simulink library "LUT_Susp_Lib"  (R2023b)
settings: Solver=VariableStepAuto  StartTime=0.0  StopTime=10.0  RelTol=1e-3
undefined symbols (not defined in the file or in its folder): Compliance, hp_wheel_ctr, JUnsprungMass, mUnsprungMass, spring_f, spring_x, Susp, Visual
libraries: nesl_utility x12, sm_lib x5, linkage_bushing_6DOF_lib x1
settings Model: Creator=smiller  LastModifiedBy=smiller
settings RTWCC: GPUComputeCapability=5.0

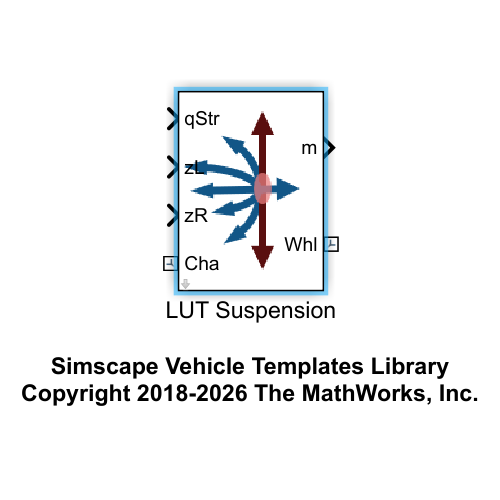
[thumbnail: Simulink's stored preview of the top-level diagram]
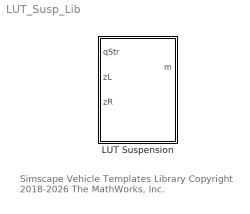
== system LUT_Susp_Lib ==
  note: Simscape Vehicle Templates Library
      | Copyright 2018-2026 The MathWorks, Inc.
  LUT Suspension : Subsystem  mask(Lookup-Table Based Suspension){popup_leftRight=Left, kin_qz_vec=Susp.LUT.Kinematics.aToe.Value, kin_zvec_qz=Susp.LUT.Kinematics.zaToe.Value, kin_qvec_qz=Susp.LUT.Kinematics.qaToe.Value, kin_qy_vec=Susp.LUT.Kinematics.aCaster.Value, kin_zvec_qy=Susp.LUT.Kinematics.zaCaster.Value, kin_qvec_qy=Susp.LUT.Kinematics.qaCaster.Value, kin_qx_vec=Susp.LUT.Kinematics.aCamber.Value, kin_zvec_qx=Susp.LUT.Kinematics.zaCamber.Value, kin_qvec_qx=Susp.LUT.Kinematics.qaCamber.Value, kin_px_vec=Susp.LUT.Kinematics.xLong.Value, kin_zvec_px=Susp.LUT.Kinematics.zxLong.Value, kin_qvec_px=Susp.LUT.Kinematics.qxLong.Value, kin_py_vec=Susp.LUT.Kinematics.xLat.Value, kin_zvec_py=Susp.LUT.Kinematics.zxLat.Value, kin_qvec_py=Susp.LUT.Kinematics.qxLat.Value, kin_fz_vec=spring_f, kin_zvec_fz=spring_x, kin_vr_vec=Susp.LUT.Spring.vrt.Value, kin_zvec_vr=Susp.LUT.Spring.zvrt.Value, spring_b=5500, kin_arbfz_vec=Susp.LUT.AntiRollBar.f.Value, kin_dzvec_arbfz=Susp.LUT.AntiRollBar.dz.Value, kin_tFilt=1e-3, tFilt_pz=1e-3, Compliance=Compliance, checkbox_setTargets=on, shell_or=Visual.hp.rad*2, elastomer_ir=Visual.hp.rad, shell_len=Visual.hp.rad*2, elastomer_clr=Visual.Bushing.clr, elastomer_opc=Visual.part.opc, elastomer_axis_clr=Visual.BushingXAxis.clr, mUnsprungMass=mUnsprungMass, JUnsprungMass=JUnsprungMass}
      mask prompts: popup_leftRight "Left/Right"; spring_b "Damping (N/(m/s))"; kin_arbfz_vec "Anti Roll Bar Force (N)"; kin_dzvec_arbfz "Wheel Center Height Difference (L-R) (m)"; kin_tFilt "Filter Time Constant Kinematics (s)"; tFilt_pz "Filter Time Constant, Height (s)"; checkbox_setTargets "Set position targets to 0"; shell_or "Shell Outer Radius (m)"; elastomer_ir "Elastomer Inner Radius (m)"; shell_len "Shell Length (m)"; elastomer_clr "Elastomer Color [R G B]"; elastomer_opc "Elastomer Opacity [R G B]"; elastomer_axis_clr "Elastomer Axis Color [R G B]"; mUnsprungMass "Mass (kg)"; JUnsprungMass "Inertia (kg*m^2)"
      mask help: Abstract car suspension based on lookup tables. The wheel frame lateral position. longitudinal position, and orientation are defined based on lookup tables that use the wheel frame height and steering wheel angle as an input. A spring-damper is included that acts along the vertical degree of freedom. The spring-damper force is based on lookup tables that capture spring stiffness, damping, and the anti-roll bar. An optional compliance element is defined at the wheel frame with 6 degrees of freedom.
      mask init:
      | curblk = gcb;
      | 
      | if(popup_leftRight==1)
      |     rhs = 1;
      | %    set_param([curblk '/Revolute Steer'],'popup_leftRight','Left')
      | else
      |     rhs = -1;
      | %    set_param([curblk '/Revolute Steer'],'popup_leftRight','Right')
      | end
      | 
      | %compOpt = get_param(curblk,'popup_compliance');
      | %set_param([curblk '/Compliance'],'LabelModeActiveChoice',compOpt);
      | 
      | %{
      | set_param([curblk '/Compliance/Bushing'],...
      |     'checkbox_setTargets',checkbox_setTargets,...
      |     'popup_force_law_spr_axiX',get_param(curblk,'popup_force_law_spr_axiX'),...
      |     'popup_force_law_spr_axiY',get_param(curblk,'popup_force_law_spr_axiY'),...
      |     'popup_force_law_spr_axiZ',get_param(curblk,'popup_force_law_spr_axiZ'),...
      |     'popup_force_law_dam_axiX',get_param(curblk,'popup_force_law_dam_axiX'),...
      |     'popup_force_law_dam_axiY',get_param(curblk,'popup_force_law_dam_axiY'),...
      |     'popup_force_law_dam_axiZ',get_param(curblk,'popup_force_law_dam_axiZ'),...
      |     'popup_force_law_spr_torX',get_param(curblk,'popup_force_law_spr_torX'),...
      |     'popup_force_law_spr_torY',get_param(curblk,'popup_force_law_spr_torY'),...
      |     'popup_force_law_spr_torZ',get_param(curblk,'popup_force_law_spr_torZ'),...
      |     'popup_force_law_dam_torX',get_param(curblk,'popup_force_law_dam_torX'),...
      |     'popup_force_law_dam_torY',get_param(curblk,'popup_force_law_dam_torY'),...
      |     'popup_force_law_dam_torZ',get_param(curblk,'popup_force_law_dam_torZ')...
      |     );
      | %}
      mask TypeOptions popup_leftRight: Left | Right
      mask TypeOptions kin_qz_vec: Kinematic/kin_qz_vec
      mask TypeOptions kin_zvec_qz: Kinematic/kin_zvec_qz
      mask TypeOptions kin_qvec_qz: Kinematic/kin_qvec_qz
      mask TypeOptions kin_qy_vec: Kinematic/kin_qy_vec
      mask TypeOptions kin_zvec_qy: Kinematic/kin_zvec_qy
      mask TypeOptions kin_qvec_qy: Kinematic/kin_qvec_qy
      mask TypeOptions kin_qx_vec: Kinematic/kin_qx_vec
      mask TypeOptions kin_zvec_qx: Kinematic/kin_zvec_qx
      mask TypeOptions kin_qvec_qx: Kinematic/kin_qvec_qx
      mask TypeOptions kin_px_vec: Kinematic/kin_px_vec
      mask TypeOptions kin_zvec_px: Kinematic/kin_zvec_px
      mask TypeOptions kin_qvec_px: Kinematic/kin_qvec_px
      mask TypeOptions kin_py_vec: Kinematic/kin_py_vec
      mask TypeOptions kin_zvec_py: Kinematic/kin_zvec_py
      mask TypeOptions kin_qvec_py: Kinematic/kin_qvec_py
      mask TypeOptions kin_fz_vec: Kinematic/kin_fz_vec
      mask TypeOptions kin_zvec_fz: Kinematic/kin_zvec_fz
      mask TypeOptions kin_vr_vec: Kinematic/kin_vr_vec
      mask TypeOptions kin_zvec_vr: Kinematic/kin_zvec_vr
      mask TypeOptions spring_b: Kinematic/spring_b
      mask TypeOptions kin_arbfz_vec: Kinematic/kin_arbfz_vec
      mask TypeOptions kin_dzvec_arbfz: Kinematic/kin_dzvec_arbfz
      mask TypeOptions kin_tFilt: Kinematic/kin_tFilt
      mask TypeOptions tFilt_pz: Kinematic/tFilt_pz
      mask DialogControl cont_kinematics Prompt: Kinematics
      mask DialogControl text_kin_value Prompt: Value
      mask DialogControl text_kin_height Prompt: Height (m)
      mask DialogControl text_kin_steer Prompt: Steer Angle (rad)
      mask DialogControl text_kin_zvec_qz Prompt: Toe Angle (deg)
      mask DialogControl text_kin_qy_vec Prompt: Caster Angle (deg)
      mask DialogControl text_kin_qx_vec Prompt: Camber Angle (deg)
      mask DialogControl text_kin_px_vec Prompt: Longitud. Pos. (m)
      mask DialogControl text_kin_py_vec Prompt: Lateral Position (m)
      mask DialogControl text_kin_fz_vec Prompt: Spring Force (N)
      mask DialogControl text_kin_vr_vec Prompt: Velocity Ratio (1)
      mask DialogControl cont_arb Prompt: Anti Roll Bar
      mask DialogControl cont_cpl Prompt: Compliance
      mask DialogControl cont_vis Prompt: Visualization
      mask DialogControl cont_dim Prompt: Unsprung Mass
      mask Display: image('sm_car_vehicle_susp_lutL_IMAGE.png')

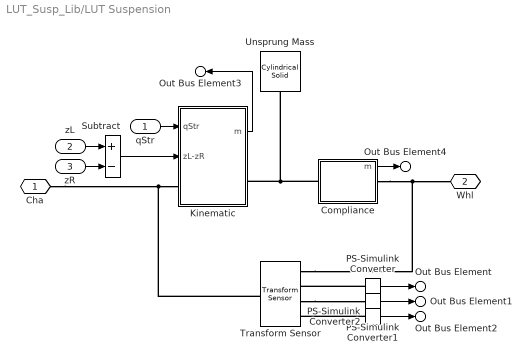
== system LUT_Susp_Lib/LUT Suspension ==
  qStr : Inport
  zL : Inport  Port=2
  zR : Inport  Port=3
  Compliance : Subsystem  Variant=on  VariantControlMode=label  VariantControl=Bushing  LabelModeActiveChoice=Rigid  mask(Optional Compliance){Connection=Compliance, VariantLabel=Compliance.class.Value}
      mask prompts: Connection "Connection Parameters"; VariantLabel "Variant Label"
      mask help: Optional compliance. Includes all 6 degrees of freedom, force laws can be linear or table. Parameters are passed in via a structure. To omit compliance set Variant Label to 'Rigid'.
      mask init:
      | curblk = gcb;
      | 
      | % Set variant for this block 
      | set_param(curblk,'LabelModeActiveChoice',VariantLabel);
  Kinematic : Subsystem  mask(Suspension with Lookup-Table Based Constraints){kin_tFilt=kin_tFilt, tFilt_pz=tFilt_pz, spring_b=spring_b, rhs_val=rhs, kin_qz_vec=kin_qz_vec, kin_zvec_qz=kin_zvec_qz, kin_qvec_qz=kin_qvec_qz, kin_qy_vec=kin_qy_vec, kin_zvec_qy=kin_zvec_qy, kin_qvec_qy=kin_qvec_qy, kin_qx_vec=kin_qx_vec, kin_zvec_qx=kin_zvec_qx, kin_qvec_qx=kin_qvec_qx, kin_px_vec=kin_px_vec, kin_zvec_px=kin_zvec_px, kin_qvec_px=kin_qvec_px, kin_py_vec=kin_py_vec, kin_zvec_py=kin_zvec_py, kin_qvec_py=kin_qvec_py, kin_fz_vec=kin_fz_vec, kin_zvec_fz=kin_zvec_fz, kin_vr_vec=kin_vr_vec, kin_zvec_vr=kin_zvec_vr, kin_dzvec_arbfz=kin_dzvec_arbfz, kin_arbfz_vec=kin_arbfz_vec}
      mask prompts: kin_tFilt "Filter Time Constant, Kinematics (s)"; tFilt_pz "Filter Time Constant, Height (s)"; spring_b "Damping (N/m/s))"; rhs_val "Left (1) or Right (-1)"; kin_dzvec_arbfz "Wheel Center Height Difference (L-R) (m)"; kin_arbfz_vec "ARB Force (N)"
      mask help: Models constraints required for lookup-table based kinematic suspension. The wheel frame lateral position, longitudinal position, and orientation are defined based on lookup tables that use the wheel frame height and steering wheel angle as an input. A spring-damper is included that acts along the vertical degree of freedom. The spring-damper force is based on lookup tables that capture spring stiffness, damping, and the anti-roll bar.
      mask TypeOptions spring_b: Spring Damper/spring_b
      mask TypeOptions kin_fz_vec: Spring Damper/kin_fz_vec
      mask TypeOptions kin_zvec_fz: Spring Damper/kin_zvec_fz
      mask TypeOptions kin_vr_vec: Spring Damper/kin_vr_vec
      mask TypeOptions kin_zvec_vr: Spring Damper/kin_zvec_vr
      mask TypeOptions kin_dzvec_arbfz: Spring Damper/kin_dzvec_arbfz
      mask TypeOptions kin_arbfz_vec: Spring Damper/kin_arbfz_vec
      mask DialogControl cont_kinematics Prompt: Kinematics
      mask DialogControl text_kin_value Prompt: Value
      mask DialogControl text_kin_height Prompt: Height (m)
      mask DialogControl text_kin_steer Prompt: Steer (rad)
      mask DialogControl text_kin_zvec_qz Prompt: Toe Angle (deg)
      mask DialogControl text_kin_qy_vec Prompt: Caster Angle (deg)
      mask DialogControl text_kin_qx_vec Prompt: Camber Angle (deg)
      mask DialogControl text_kin_px_vec Prompt: Longitud. Pos. (m)
      mask DialogControl text_kin_py_vec Prompt: Lateral Position (m)
      mask DialogControl text_kin_fz_vec Prompt: Spring Force (N)
      mask DialogControl text_kin_vr_vec_copy Prompt: Velocity Ratio (1)
      mask DialogControl cont_arb Prompt: Anti Roll Bar
  PS-Simulink Converter : nesl_utility/PS-Simulink Converter  PhysicalDomain=network_engine_domain  SubClassName=ps_output  LeftPortType=input  RightPortType=output  PseudoPeriodic=off  Frequencies=[]  VectorFormat=inherit  Unit=inherit  AffineConversion=off
  PS-Simulink Converter1 : nesl_utility/PS-Simulink Converter  PhysicalDomain=network_engine_domain  SubClassName=ps_output  LeftPortType=input  RightPortType=output  PseudoPeriodic=off  Frequencies=[]  VectorFormat=inherit  Unit=inherit  AffineConversion=off
  PS-Simulink Converter2 : nesl_utility/PS-Simulink Converter  PhysicalDomain=network_engine_domain  SubClassName=ps_output  LeftPortType=input  RightPortType=output  PseudoPeriodic=off  Frequencies=[]  VectorFormat=inherit  Unit=inherit  AffineConversion=off
  Subtract : Sum  Inputs=+-
  Transform Sensor : sm_lib/Frames and Transforms/Transform Sensor  MeasurementFrame=Base  RotationSequence=XYX  SenseAngle=off  SenseAxis=off  SenseQ=off  SenseR=off  SenseRotationSequence=off  SenseOmegaX=off  SenseOmegaY=off  SenseOmegaZ=off  SenseOmega=off  SenseQDot=off  SenseRDot=off  SenseRotationSequenceDot=off  SenseAlphaX=off  SenseAlphaY=off  SenseAlphaZ=off  SenseAlpha=off  SenseQDDot=off  SenseRDDot=off  SenseX=on  SenseY=on  SenseZ=on  SenseXYZ=off  SenseRad=off  SenseAzim=off  SenseDist=off  SenseInc=off  SenseXDot=off  SenseYDot=off  SenseZDot=off  SenseXYZDot=off  SenseRadDot=off  SenseAzimDot=off  SenseDistDot=off  SenseIncDot=off  SenseXDDot=off  SenseYDDot=off  SenseZDDot=off  SenseXYZDDot=off  SenseRadDDot=off  SenseAzimDDot=off  SenseDistDDot=off  SenseIncDDot=off
  Unsprung Mass : sm_lib/Body Elements/Cylindrical Solid  GraphicAmbientColor=[0.15 0.15 0.15 1.0]  BasedOnType=Density  CenterOfMass=[0 0 0]  CenterOfMassUnits=m  GraphicDiffuseColor=[0.07451 0.6235 1]  CylinderLength=1e-2  CylinderLengthUnits=m  CylinderRadius=1e-2  CylinderRadiusUnits=m  Density=1000  DensityUnits=kg/m^3  DoExposeReferenceFrame=on  GraphicEmissiveColor=[0.0 0.0 0.0 1.0]  ExportEntireGeometry=off  SerializedFrames=<Frames/>  MarkerShape=Sphere  MarkerSize=10  GraphicType=FromGeometry  InertiaType=Custom  Mass=mUnsprungMass  MassUnits=kg  MomentsOfInertia=JUnsprungMass  MomentsOfInertiaUnits=kg*m^2  GraphicOpacity=1  ProductsOfInertia=[0 0 0]  ProductsOfInertiaUnits=kg*m^2  GraphicShininess=75  GraphicSpecularColor=[0.5 0.5 0.5 1.0]  GraphicVisPropType=SimpleVisualProperties
  Cha : PMIOPort  Side=Left
  Whl : PMIOPort  Port=2  Side=Right
  Out Bus Element : Outport  PortName=m  Element=px
  Out Bus Element1 : Outport  PortName=m  Element=py
  Out Bus Element2 : Outport  PortName=m  Element=pz
  Out Bus Element3 : Outport  PortName=m  Element=Kinematic
  Out Bus Element4 : Outport  PortName=m  Element=Compliance
  wires:
  qStr/1 -> Kinematic/1(qStr)
  PS-Simulink Converter/1 -> Out Bus Element/1
  PS-Simulink Converter1/1 -> Out Bus Element1/1
  PS-Simulink Converter2/1 -> Out Bus Element2/1
  Kinematic/1(m) -> Out Bus Element3/1
  zL/1 -> Subtract/1
  zR/1 -> Subtract/2
  Subtract/1 -> Kinematic/2(zL-zR)
  Compliance/1(m) -> Out Bus Element4/1
  connections:
  Compliance/LConn1 -- Unsprung Mass/RConn1 -- Kinematic/RConn1
  Compliance/RConn1 -- Whl/RConn1 -- Transform Sensor/RConn1
  PS-Simulink Converter/LConn1 -- Transform Sensor/RConn2
  Transform Sensor/RConn3 -- PS-Simulink Converter1/LConn1
  PS-Simulink Converter2/LConn1 -- Transform Sensor/RConn4
  Transform Sensor/LConn1 -- Cha/RConn1 -- Kinematic/LConn1

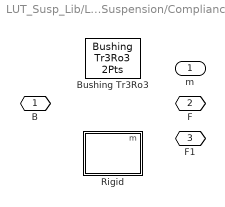
== system LUT_Susp_Lib/LUT Suspension/Compliance ==
  Bushing Tr3Ro3 : linkage_bushing_6DOF_lib/Bushing Tr3Ro3 2Pts  VariantControl=Bushing_Tr3Ro3  checkbox_setTargets=on  leftOrRight=rhs  hp_j=hp_wheel_ctr.*[1 rhs 1]  hp_z=hp_wheel_ctr.*[1 rhs 1]+[0 0 1]  hp_x=hp_wheel_ctr.*[1 rhs 1]+[1 0 0]  sprx=Connection.SpringX  spry=Connection.SpringY  sprz=Connection.SpringZ  damx=Connection.DamperX  damy=Connection.DamperY  damz=Connection.DamperZ  sprqx=Connection.SpringqX  sprqy=Connection.SpringqY  sprqz=Connection.SpringqZ  damqx=Connection.DamperqX  damqy=Connection.DamperqY  damqz=Connection.DamperqZ  shell_or=Visual.hp.rad*2  shell_len=Visual.hp.rad*2  shell_clr=Visual.BushingShell.clr  shell_opc=Visual.part.opc  sleeve_clr=Visual.Bushing.clr  sleeve_opc=Visual.part.opc
  Rigid : Subsystem  VariantControl=Rigid
  B : PMIOPort  Side=Left
  F : PMIOPort  Port=2  Side=Right
  F1 : PMIOPort  Port=3  Side=Right
  m : Outport

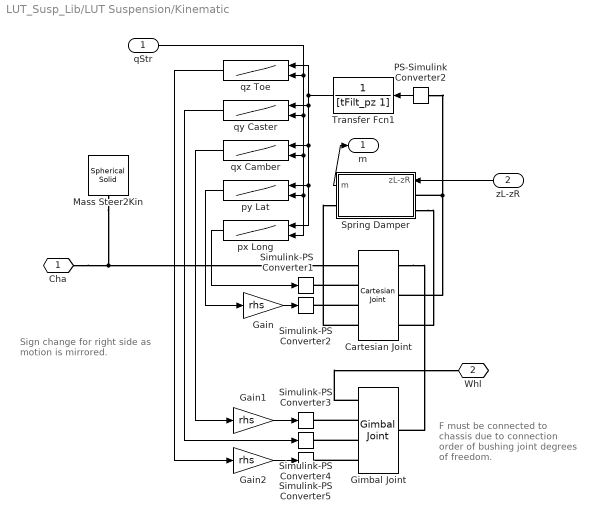
== system LUT_Susp_Lib/LUT Suspension/Kinematic ==
  note: Sign change for right side as motion is mirrored.
  note: F must be connected to chassis due to connection order of bushing joint degrees of freedom.
  qStr : Inport
  zL-zR : Inport  Port=2
  Cartesian Joint : sm_lib/Joints/Cartesian Joint  JointMode=Normal  SenseConstraintForce=off  SenseConstraintForceX=off  SenseConstraintForceY=off  SenseConstraintForceZ=off  SenseConstraintTorque=off  SenseConstraintTorqueX=off  SenseConstraintTorqueY=off  SenseConstraintTorqueZ=off  SenseTotalForce=off  SenseTotalForceX=off  SenseTotalForceY=off  SenseTotalForceZ=off  SenseTotalTorque=off  SenseTotalTorqueX=off  SenseTotalTorqueY=off  SenseTotalTorqueZ=off  CompositeWrenchDir=FollowerOnBase  CompositeWrenchFrame=BaseFrame  PxEquilibriumPosition=0  PxEquilibriumPositionUnits=m  PxSpringStiffness=0  PxSpringStiffnessUnits=N/m  PxDampingCoefficient=0  PxDampingCoefficientUnits=N/(m/s)  PxTorqueActuationMode=ComputedTorque  PxMotionActuationMode=InputMotion  PxSensePosition=off  PxSenseVelocity=off  PxSenseAcceleration=off  PxSenseTorqueForce=off  PxSenseLowerLimitTorqueForce=off  PxSenseUpperLimitTorqueForce=off  PxLowerLimitSpecify=off  PxLowerLimitBound=-1  PxLowerLimitBoundUnits=m  PxLowerLimitStiffness=1e6  PxLowerLimitStiffnessUnits=N/m  PxLowerLimitDamping=1e3  PxLowerLimitDampingUnits=N/(m/s)  PxLowerLimitTransitionRegionWidth=1e-4  PxLowerLimitTransitionRegionWidthUnits=m  PxUpperLimitSpecify=off  PxUpperLimitBound=1  PxUpperLimitBoundUnits=m  PxUpperLimitStiffness=1e6  PxUpperLimitStiffnessUnits=N/m  PxUpperLimitDamping=1e3  PxUpperLimitDampingUnits=N/(m/s)  PxUpperLimitTransitionRegionWidth=1e-4  PxUpperLimitTransitionRegionWidthUnits=m  PxPositionTargetSpecify=on  PxPositionTargetPriority=Low  PxPositionTargetValue=0  PxPositionTargetValueUnits=m  PxVelocityTargetSpecify=off  PxVelocityTargetPriority=High  PxVelocityTargetValue=0  PxVelocityTargetValueUnits=m/s  PyEquilibriumPosition=0  PyEquilibriumPositionUnits=m  PySpringStiffness=0  PySpringStiffnessUnits=N/m  PyDampingCoefficient=0  PyDampingCoefficientUnits=N/(m/s)  PyTorqueActuationMode=ComputedTorque  PyMotionActuationMode=InputMotion  PySensePosition=off  PySenseVelocity=off  PySenseAcceleration=off  PySenseTorqueForce=off  PySenseLowerLimitTorqueForce=off  PySenseUpperLimitTorqueForce=off  PyLowerLimitSpecify=off  PyLowerLimitBound=-1  PyLowerLimitBoundUnits=m  PyLowerLimitStiffness=1e6  PyLowerLimitStiffnessUnits=N/m  PyLowerLimitDamping=1e3  PyLowerLimitDampingUnits=N/(m/s)  PyLowerLimitTransitionRegionWidth=1e-4  PyLowerLimitTransitionRegionWidthUnits=m  PyUpperLimitSpecify=off  PyUpperLimitBound=1  PyUpperLimitBoundUnits=m  PyUpperLimitStiffness=1e6  PyUpperLimitStiffnessUnits=N/m  PyUpperLimitDamping=1e3  PyUpperLimitDampingUnits=N/(m/s)  PyUpperLimitTransitionRegionWidth=1e-4  PyUpperLimitTransitionRegionWidthUnits=m  PyPositionTargetSpecify=on  PyPositionTargetPriority=Low  PyPositionTargetValue=0  PyPositionTargetValueUnits=m  PyVelocityTargetSpecify=off  PyVelocityTargetPriority=High  PyVelocityTargetValue=0  PyVelocityTargetValueUnits=m/s  PzEquilibriumPosition=0  PzEquilibriumPositionUnits=m  PzSpringStiffness=0  PzSpringStiffnessUnits=N/m  PzDampingCoefficient=0  PzDampingCoefficientUnits=N/(m/s)  PzTorqueActuationMode=InputTorque  PzMotionActuationMode=ComputedMotion  PzSensePosition=on  PzSenseVelocity=on  PzSenseAcceleration=off  PzSenseTorqueForce=off  PzSenseLowerLimitTorqueForce=off  PzSenseUpperLimitTorqueForce=off  PzLowerLimitSpecify=off  PzLowerLimitBound=-1  PzLowerLimitBoundUnits=m  PzLowerLimitStiffness=1e6  PzLowerLimitStiffnessUnits=N/m  PzLowerLimitDamping=1e3  PzLowerLimitDampingUnits=N/(m/s)  PzLowerLimitTransitionRegionWidth=1e-4  PzLowerLimitTransitionRegionWidthUnits=m  PzUpperLimitSpecify=off  PzUpperLimitBound=1  PzUpperLimitBoundUnits=m  PzUpperLimitStiffness=1e6  PzUpperLimitStiffnessUnits=N/m  PzUpperLimitDamping=1e3  PzUpperLimitDampingUnits=N/(m/s)  PzUpperLimitTransitionRegionWidth=1e-4  PzUpperLimitTransitionRegionWidthUnits=m  PzPositionTargetSpecify=on  PzPositionTargetPriority=Low  PzPositionTargetValue=0  PzPositionTargetValueUnits=m  PzVelocityTargetSpecify=off  PzVelocityTargetPriority=High  PzVelocityTargetValue=0  PzVelocityTargetValueUnits=m/s
  Gain : Gain  Gain=rhs
  Gain1 : Gain  Gain=rhs
  Gain2 : Gain  Gain=rhs
  Gimbal Joint : sm_lib/Joints/Gimbal Joint  JointMode=Normal  SenseConstraintForce=off  SenseConstraintForceX=off  SenseConstraintForceY=off  SenseConstraintForceZ=off  SenseConstraintTorque=off  SenseConstraintTorqueX=off  SenseConstraintTorqueY=off  SenseConstraintTorqueZ=off  SenseTotalForce=off  SenseTotalForceX=off  SenseTotalForceY=off  SenseTotalForceZ=off  SenseTotalTorque=off  SenseTotalTorqueX=off  SenseTotalTorqueY=off  SenseTotalTorqueZ=off  CompositeWrenchDir=FollowerOnBase  CompositeWrenchFrame=BaseFrame  RxEquilibriumPosition=0  RxEquilibriumPositionUnits=deg  RxSpringStiffness=0  RxSpringStiffnessUnits=N*m/deg  RxDampingCoefficient=0  RxDampingCoefficientUnits=N*m/(deg/s)  RxTorqueActuationMode=ComputedTorque  RxMotionActuationMode=InputMotion  RxSensePosition=off  RxSenseVelocity=off  RxSenseAcceleration=off  RxSenseTorqueForce=off  RxSenseLowerLimitTorqueForce=off  RxSenseUpperLimitTorqueForce=off  RxLowerLimitSpecify=off  RxLowerLimitBound=-90  RxLowerLimitBoundUnits=deg  RxLowerLimitStiffness=1e4  RxLowerLimitStiffnessUnits=N*m/deg  RxLowerLimitDamping=10  RxLowerLimitDampingUnits=N*m/(deg/s)  RxLowerLimitTransitionRegionWidth=0.1  RxLowerLimitTransitionRegionWidthUnits=deg  RxUpperLimitSpecify=off  RxUpperLimitBound=90  RxUpperLimitBoundUnits=deg  RxUpperLimitStiffness=1e4  RxUpperLimitStiffnessUnits=N*m/deg  RxUpperLimitDamping=10  RxUpperLimitDampingUnits=N*m/(deg/s)  RxUpperLimitTransitionRegionWidth=0.1  RxUpperLimitTransitionRegionWidthUnits=deg  RxPositionTargetSpecify=on  RxPositionTargetPriority=Low  RxPositionTargetValue=0  RxPositionTargetValueUnits=deg  RxVelocityTargetSpecify=off  RxVelocityTargetPriority=High  RxVelocityTargetValue=0  RxVelocityTargetValueUnits=deg/s  RyEquilibriumPosition=0  RyEquilibriumPositionUnits=deg  RySpringStiffness=0  RySpringStiffnessUnits=N*m/deg  RyDampingCoefficient=0  RyDampingCoefficientUnits=N*m/(deg/s)  RyTorqueActuationMode=ComputedTorque  RyMotionActuationMode=InputMotion  RySensePosition=off  RySenseVelocity=off  RySenseAcceleration=off  RySenseTorqueForce=off  RySenseLowerLimitTorqueForce=off  RySenseUpperLimitTorqueForce=off  RyLowerLimitSpecify=off  RyLowerLimitBound=-90  RyLowerLimitBoundUnits=deg  RyLowerLimitStiffness=1e4  RyLowerLimitStiffnessUnits=N*m/deg  RyLowerLimitDamping=10  RyLowerLimitDampingUnits=N*m/(deg/s)  RyLowerLimitTransitionRegionWidth=0.1  RyLowerLimitTransitionRegionWidthUnits=deg  RyUpperLimitSpecify=off  RyUpperLimitBound=90  RyUpperLimitBoundUnits=deg  RyUpperLimitStiffness=1e4  RyUpperLimitStiffnessUnits=N*m/deg  RyUpperLimitDamping=10  RyUpperLimitDampingUnits=N*m/(deg/s)  RyUpperLimitTransitionRegionWidth=0.1  RyUpperLimitTransitionRegionWidthUnits=deg  RyPositionTargetSpecify=on  RyPositionTargetPriority=Low  RyPositionTargetValue=0  RyPositionTargetValueUnits=deg  RyVelocityTargetSpecify=off  RyVelocityTargetPriority=High  RyVelocityTargetValue=0  RyVelocityTargetValueUnits=deg/s  RzEquilibriumPosition=0  RzEquilibriumPositionUnits=deg  RzSpringStiffness=0  RzSpringStiffnessUnits=N*m/deg  RzDampingCoefficient=0  RzDampingCoefficientUnits=N*m/(deg/s)  RzTorqueActuationMode=ComputedTorque  RzMotionActuationMode=InputMotion  RzSensePosition=off  RzSenseVelocity=off  RzSenseAcceleration=off  RzSenseTorqueForce=off  RzSenseLowerLimitTorqueForce=off  RzSenseUpperLimitTorqueForce=off  RzLowerLimitSpecify=off  RzLowerLimitBound=-90  RzLowerLimitBoundUnits=deg  RzLowerLimitStiffness=1e4  RzLowerLimitStiffnessUnits=N*m/deg  RzLowerLimitDamping=10  RzLowerLimitDampingUnits=N*m/(deg/s)  RzLowerLimitTransitionRegionWidth=0.1  RzLowerLimitTransitionRegionWidthUnits=deg  RzUpperLimitSpecify=off  RzUpperLimitBound=90  RzUpperLimitBoundUnits=deg  RzUpperLimitStiffness=1e4  RzUpperLimitStiffnessUnits=N*m/deg  RzUpperLimitDamping=10  RzUpperLimitDampingUnits=N*m/(deg/s)  RzUpperLimitTransitionRegionWidth=0.1  RzUpperLimitTransitionRegionWidthUnits=deg  RzPositionTargetSpecify=on  RzPositionTargetPriority=Low  RzPositionTargetValue=0  RzPositionTargetValueUnits=deg  RzVelocityTargetSpecify=off  RzVelocityTargetPriority=High  RzVelocityTargetValue=0  RzVelocityTargetValueUnits=deg/s
  Mass Steer2Kin : sm_lib/Body Elements/Spherical Solid  GraphicAmbientColor=[0.15 0.15 0.15 1.0]  BasedOnType=Density  CenterOfMass=[0 0 0]  CenterOfMassUnits=m  GraphicDiffuseColor=[0.5 0.5 0.5]  Density=1000  DensityUnits=kg/m^3  DoExposeReferenceFrame=on  GraphicEmissiveColor=[0.0 0.0 0.0 1.0]  ExportEntireGeometry=off  SerializedExposedGeometries=<ExposedGeometries/>  SerializedFrames=<Frames/>  MarkerShape=Sphere  MarkerSize=10  GraphicType=FromGeometry  InertiaType=CalculateFromGeometry  Mass=1  MassUnits=kg  MomentsOfInertia=[1 1 1]  MomentsOfInertiaUnits=kg*m^2  GraphicOpacity=1  ProductsOfInertia=[0 0 0]  ProductsOfInertiaUnits=kg*m^2  GraphicShininess=75  GraphicSpecularColor=[0.5 0.5 0.5 1.0]  SphereRadius=1e-3  SphereRadiusUnits=m  GraphicVisPropType=SimpleVisualProperties
  PS-Simulink Converter2 : nesl_utility/PS-Simulink Converter  PhysicalDomain=network_engine_domain  SubClassName=ps_output  LeftPortType=input  RightPortType=output  PseudoPeriodic=off  Frequencies=[]  VectorFormat=inherit  Unit=inherit  AffineConversion=off
  Simulink-PS Converter1 : nesl_utility/Simulink-PS Converter  PhysicalDomain=network_engine_domain  SubClassName=ps_input  LeftPortType=input  RightPortType=output  PseudoPeriodic=off  Frequencies=[]  NoiseDistribution=none  NoiseParameters=[]  Unit=m  AffineConversion=off  FilteringAndDerivatives=filter  SimscapeFilterOrder=2  InputFilterTimeConstant=kin_tFilt  UdotUserProvided=0
  Simulink-PS Converter2 : nesl_utility/Simulink-PS Converter  PhysicalDomain=network_engine_domain  SubClassName=ps_input  LeftPortType=input  RightPortType=output  PseudoPeriodic=off  Frequencies=[]  NoiseDistribution=none  NoiseParameters=[]  Unit=m  AffineConversion=off  FilteringAndDerivatives=filter  SimscapeFilterOrder=2  InputFilterTimeConstant=kin_tFilt  UdotUserProvided=0
  Simulink-PS Converter3 : nesl_utility/Simulink-PS Converter  PhysicalDomain=network_engine_domain  SubClassName=ps_input  LeftPortType=input  RightPortType=output  PseudoPeriodic=off  Frequencies=[]  NoiseDistribution=none  NoiseParameters=[]  Unit=deg  AffineConversion=off  FilteringAndDerivatives=filter  SimscapeFilterOrder=2  InputFilterTimeConstant=kin_tFilt  UdotUserProvided=0
  Simulink-PS Converter4 : nesl_utility/Simulink-PS Converter  PhysicalDomain=network_engine_domain  SubClassName=ps_input  LeftPortType=input  RightPortType=output  PseudoPeriodic=off  Frequencies=[]  NoiseDistribution=none  NoiseParameters=[]  Unit=deg  AffineConversion=off  FilteringAndDerivatives=filter  SimscapeFilterOrder=2  InputFilterTimeConstant=kin_tFilt  UdotUserProvided=0
  Simulink-PS Converter5 : nesl_utility/Simulink-PS Converter  PhysicalDomain=network_engine_domain  SubClassName=ps_input  LeftPortType=input  RightPortType=output  PseudoPeriodic=off  Frequencies=[]  NoiseDistribution=none  NoiseParameters=[]  Unit=deg  AffineConversion=off  FilteringAndDerivatives=filter  SimscapeFilterOrder=2  InputFilterTimeConstant=kin_tFilt  UdotUserProvided=0
  Spring Damper : Subsystem  mask(Spring Damper Force){rhs=rhs, spring_b=spring_b, kin_fz_vec=kin_fz_vec, kin_zvec_fz=kin_zvec_fz, kin_vr_vec=kin_vr_vec, kin_zvec_vr=kin_zvec_vr, kin_arbfz_vec=kin_arbfz_vec, kin_dzvec_arbfz=kin_dzvec_arbfz}
      mask prompts: rhs "Left (1) or Right (-1)"; spring_b "Damping (N/m/s))"; kin_fz_vec "Spring Force (N)"; kin_zvec_fz "Wheel Center Height (m)"; kin_vr_vec "Velocity Ratio (1)"; kin_zvec_vr "Wheel Center Height (m)"; kin_arbfz_vec "Anti Roll Bar Force (N)"; kin_dzvec_arbfz "Height Difference (L-R) (m)"
      mask help: Models a spring-damper force. Spring force is defined as a lookup table based on height. Preload is the force when the deflection is 0. Damping is single damping coefficient, and the velocity ratio scales the wheel center vertical motion to match the damper compression in the original system. The anti-roll bar lookup table defines the force couple on the left and right wheel centers due to the anti-roll bar alone.
      mask TypeOptions spring_b: Damping/Gain
      mask DialogControl Container3 Prompt: Anti Roll Bar
  Transfer Fcn1 : TransferFcn  Denominator=[tFilt_pz 1]
  px Long : Lookup_n-D  BreakpointsForDimension1=kin_zvec_px  BreakpointsForDimension2=kin_qvec_px  Table=kin_px_vec  InternalRulePriority=Speed  RndMeth=Simplest
      settings: InputPortMap=u0,u1
  py Lat : Lookup_n-D  BreakpointsForDimension1=kin_zvec_py  BreakpointsForDimension2=kin_qvec_py  Table=kin_py_vec  InternalRulePriority=Speed  RndMeth=Simplest
      settings: InputPortMap=u0,u1
  qx Camber : Lookup_n-D  BreakpointsForDimension1=kin_zvec_qx  BreakpointsForDimension2=kin_qvec_qx  Table=kin_qx_vec  InternalRulePriority=Speed  RndMeth=Simplest
      settings: InputPortMap=u0,u1
  qy Caster : Lookup_n-D  BreakpointsForDimension1=kin_zvec_qy  BreakpointsForDimension2=kin_qvec_qy  Table=kin_qy_vec  InternalRulePriority=Speed  RndMeth=Simplest
      settings: InputPortMap=u0,u1
  qz Toe : Lookup_n-D  BreakpointsForDimension1=kin_zvec_qz  BreakpointsForDimension2=kin_qvec_qz  Table=kin_qz_vec  InternalRulePriority=Speed  RndMeth=Simplest
      settings: InputPortMap=u0,u1
  Cha : PMIOPort  Side=Left
  Whl : PMIOPort  Port=2  Side=Right
  m : Outport
  wires:
  Transfer Fcn1/1 -> px Long/1, py Lat/1, qx Camber/1, qy Caster/1, qz Toe/1
  qz Toe/1 -> Gain2/1
  qx Camber/1 -> Gain1/1
  Gain/1 -> Simulink-PS Converter2/1
  qy Caster/1 -> Simulink-PS Converter4/1
  Gain2/1 -> Simulink-PS Converter5/1
  Gain1/1 -> Simulink-PS Converter3/1
  px Long/1 -> Simulink-PS Converter1/1
  py Lat/1 -> Gain/1
  PS-Simulink Converter2/1 -> Transfer Fcn1/1
  Spring Damper/1(m) -> m/1
  qStr/1 -> px Long/2, py Lat/2, qx Camber/2, qy Caster/2, qz Toe/2
  zL-zR/1 -> Spring Damper/1(zL-zR)
  connections:
  Gimbal Joint/LConn4 -- Simulink-PS Converter5/RConn1
  Cartesian Joint/LConn3 -- Simulink-PS Converter2/RConn1
  Cartesian Joint/LConn4 -- Spring Damper/RConn1
  Spring Damper/LConn2 -- Cartesian Joint/RConn3
  PS-Simulink Converter2/LConn1 -- Cartesian Joint/RConn2 -- Spring Damper/LConn1
  Cartesian Joint/LConn2 -- Simulink-PS Converter1/RConn1
  Mass Steer2Kin/RConn1 -- Cha/RConn1 -- Cartesian Joint/LConn1
  Gimbal Joint/LConn2 -- Simulink-PS Converter3/RConn1
  Gimbal Joint/LConn3 -- Simulink-PS Converter4/RConn1
  Gimbal Joint/LConn1 -- Whl/RConn1
  Cartesian Joint/RConn1 -- Gimbal Joint/RConn1

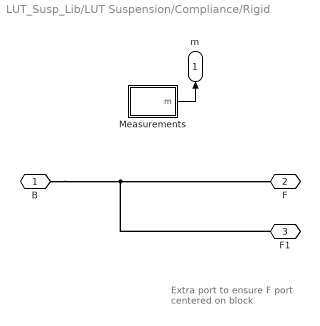
== system LUT_Susp_Lib/LUT Suspension/Compliance/Rigid ==
  note: Extra port to ensure
      | F port centered on block
  Measurements : Subsystem
  B : PMIOPort  Side=Left
  F : PMIOPort  Port=2  Side=Right
  F1 : PMIOPort  Port=3  Side=Right
  m : Outport
  wires:
  Measurements/1(m) -> m/1
  connections:
  B/RConn1 -- F1/RConn1 -- F/RConn1

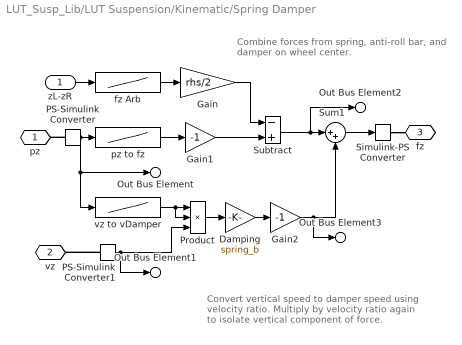
== system LUT_Susp_Lib/LUT Suspension/Kinematic/Spring Damper ==
  note: Combine forces from spring, anti-roll bar, and damper on wheel center.
  note: Convert vertical speed to damper speed using velocity ratio.
      | Multiply by velocity ratio again to isolate vertical component of force.
  zL-zR : Inport
  Damping : Gain  Gain=spring_b
  Gain : Gain  Gain=rhs/2
  Gain1 : Gain  Gain=-1
  Gain2 : Gain  Gain=-1
  PS-Simulink Converter : nesl_utility/PS-Simulink Converter  PhysicalDomain=network_engine_domain  SubClassName=ps_output  LeftPortType=input  RightPortType=output  PseudoPeriodic=off  Frequencies=[]  VectorFormat=inherit  Unit=inherit  AffineConversion=off
  PS-Simulink Converter1 : nesl_utility/PS-Simulink Converter  PhysicalDomain=network_engine_domain  SubClassName=ps_output  LeftPortType=input  RightPortType=output  PseudoPeriodic=off  Frequencies=[]  VectorFormat=inherit  Unit=inherit  AffineConversion=off
  Product : Product  Inputs=3
  Simulink-PS Converter : nesl_utility/Simulink-PS Converter  PhysicalDomain=network_engine_domain  SubClassName=ps_input  LeftPortType=input  RightPortType=output  PseudoPeriodic=off  Frequencies=[]  NoiseDistribution=none  NoiseParameters=[]  Unit=1  AffineConversion=off  FilteringAndDerivatives=provide  SimscapeFilterOrder=1  InputFilterTimeConstant=0.001  UdotUserProvided=0
  Subtract : Sum  Inputs=-+
  Sum1 : Sum  Inputs=|++
  fz Arb : Lookup_n-D  NumberOfTableDimensions=1  BreakpointsForDimension1=kin_dzvec_arbfz  Table=kin_arbfz_vec  InternalRulePriority=Speed  RndMeth=Simplest
  pz to fz : Lookup_n-D  NumberOfTableDimensions=1  BreakpointsForDimension1=kin_zvec_fz  Table=kin_fz_vec  InternalRulePriority=Speed  RndMeth=Simplest
  vz to vDamper : Lookup_n-D  NumberOfTableDimensions=1  BreakpointsForDimension1=kin_zvec_vr  Table=kin_vr_vec  InternalRulePriority=Speed  RndMeth=Simplest
  pz : PMIOPort  Side=Left
  vz : PMIOPort  Port=2  Side=Left
  fz : PMIOPort  Port=3  Side=Right
  Out Bus Element : Outport  PortName=m  Element=xSpring
  Out Bus Element1 : Outport  PortName=m  Element=vSpring
  Out Bus Element2 : Outport  PortName=m  Element=FSpring
  Out Bus Element3 : Outport  PortName=m  Element=FDamper
  wires:
  PS-Simulink Converter/1 -> vz to vDamper/1, Out Bus Element/1, pz to fz/1
  Damping/1 -> Gain2/1
  Sum1/1 -> Simulink-PS Converter/1
  pz to fz/1 -> Gain1/1
  PS-Simulink Converter1/1 -> Out Bus Element1/1, Product/3
  Subtract/1 -> Sum1/1, Out Bus Element2/1
  Gain2/1 -> Sum1/2, Out Bus Element3/1
  vz to vDamper/1 -> Product/2, Product/1
  Product/1 -> Damping/1
  zL-zR/1 -> fz Arb/1
  Gain1/1 -> Subtract/2
  fz Arb/1 -> Gain/1
  Gain/1 -> Subtract/1
  connections:
  PS-Simulink Converter/LConn1 -- pz/RConn1
  Simulink-PS Converter/RConn1 -- fz/RConn1
  PS-Simulink Converter1/LConn1 -- vz/RConn1

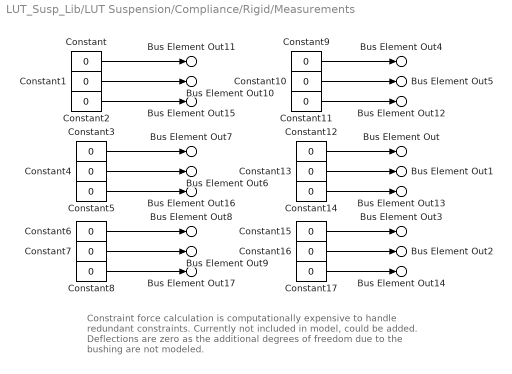
== system LUT_Susp_Lib/LUT Suspension/Compliance/Rigid/Measurements ==
  note: Constraint force calculation is computationally expensive to handle redundant constraints.  Currently not included in model, could be added.
      |
      | Deflections are zero as the additional degrees of freedom due to the bushing are not modeled.
  Constant{,1..17} (18 alike) : Constant  Value=0
  Bus Element Out : Outport  PortName=m  Element=vy
  Bus Element Out1 : Outport  PortName=m  Element=py
  Bus Element Out2 : Outport  PortName=m  Element=pz
  Bus Element Out3 : Outport  PortName=m  Element=vz
  Bus Element Out4 : Outport  PortName=m  Element=vx
  Bus Element Out5 : Outport  PortName=m  Element=px
  Bus Element Out6 : Outport  PortName=m  Element=qy
  Bus Element Out7 : Outport  PortName=m  Element=wy
  Bus Element Out8 : Outport  PortName=m  Element=wz
  Bus Element Out9 : Outport  PortName=m  Element=qz
  Bus Element Out10 : Outport  PortName=m  Element=qx
  Bus Element Out11 : Outport  PortName=m  Element=wx
  Bus Element Out12 : Outport  PortName=m  Element=fx
  Bus Element Out13 : Outport  PortName=m  Element=fy
  Bus Element Out14 : Outport  PortName=m  Element=fz
  Bus Element Out15 : Outport  PortName=m  Element=tx
  Bus Element Out16 : Outport  PortName=m  Element=ty
  Bus Element Out17 : Outport  PortName=m  Element=tz
  wires:
  Constant/1 -> Bus Element Out11/1
  Constant1/1 -> Bus Element Out10/1
  Constant2/1 -> Bus Element Out15/1
  Constant5/1 -> Bus Element Out16/1
  Constant4/1 -> Bus Element Out6/1
  Constant3/1 -> Bus Element Out7/1
  Constant8/1 -> Bus Element Out17/1
  Constant7/1 -> Bus Element Out9/1
  Constant6/1 -> Bus Element Out8/1
  Constant15/1 -> Bus Element Out3/1
  Constant16/1 -> Bus Element Out2/1
  Constant17/1 -> Bus Element Out14/1
  Constant12/1 -> Bus Element Out/1
  Constant13/1 -> Bus Element Out1/1
  Constant14/1 -> Bus Element Out13/1
  Constant11/1 -> Bus Element Out12/1
  Constant10/1 -> Bus Element Out5/1
  Constant9/1 -> Bus Element Out4/1
